simulink model "test1"  (R2017b)
settings: Solver=FixedStepAuto  StartTime=0.0  StopTime=inf  FixedStep=1e-3  RelTol=1e-3  EnableMultiTasking=on
undefined symbols (not defined in the file): D10, D11, D12, D2, D5, D8, D9, PTA0, PTA2, PTB9, PTC4, PTD0, PTD2, PTD3
libraries: frdmk64flib x12
settings Model: ExtModeTrigDuration=5  Creator=zhuh30  LastModifiedBy=Michael
settings OptimizationCC: PassReuseOutputArgsAs=Individual arguments  MaxStackSize=64
settings DebuggingCC: ParameterTunabilityLossMsg=error
settings HardwareCC: ProdBitPerPointer=32  ProdBitPerSizeT=32  ProdBitPerPtrDiffT=32  ProdLargestAtomicInteger=Long  ProdLargestAtomicFloat=Double  ProdWordSize=32  ProdHWDeviceType=ARM Compatible->ARM Cortex
settings SFSimCC: MATLABDynamicMemAlloc=off
settings RTWCC: SystemTargetFile=ert.tlc  HardwareBoard=NXP FRDM-K64F  TemplateMakefile=ert_default_tmf  GenerateReport=on  Toolchain=GNU Tools for ARM Embedded Processors  IncludeHyperlinkInReport=on  LaunchReport=on  GenerateTraceInfo=on  GenerateTraceReport=on  GenerateTraceReportSl=on  GenerateTraceReportSf=on  GenerateTraceReportEml=on
settings CodeAppCC: ForceParamTrailComments=on  IgnoreCustomStorageClasses=off  OperatorAnnotations=on  SimulinkDataObjDesc=on  SFDataObjDesc=on  InsertBlockDesc=on

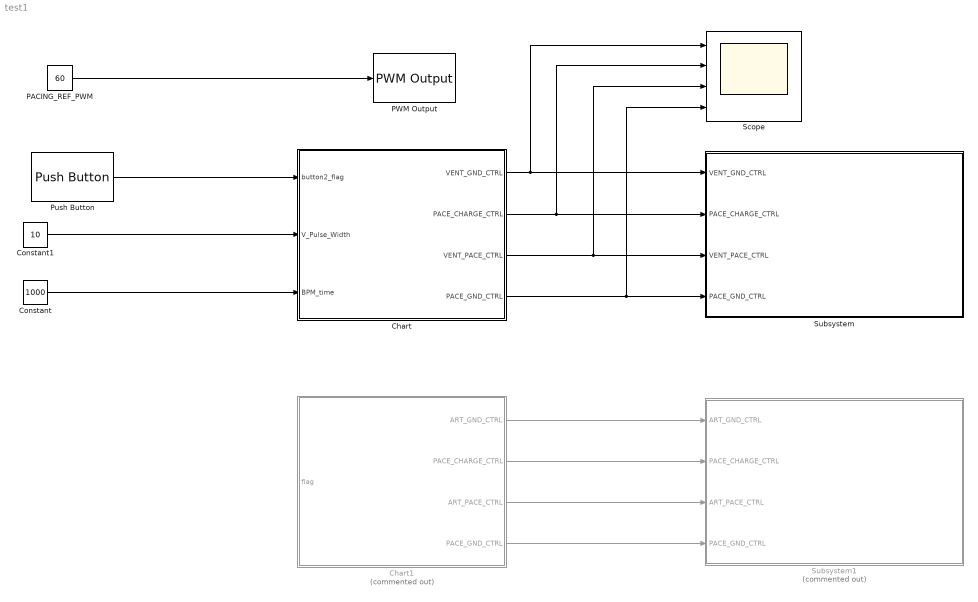
== system test1 ==
  Chart : Stateflow chart  TreatAsAtomicUnit=on
  Chart1 : Stateflow chart  Commented=on  TreatAsAtomicUnit=on
  Constant : Constant  Value=1000
  Constant1 : Constant  Value=10
  PACING_REF_PWM : Constant  Value=60  OutDataTypeStr=uint16
  PWM Output : frdmk64flib/PWM Output  Whichpin=PTA2 (D5)  InitialFrequency=1000  InitialDutyCycle=60
      settings: SourceProductName=Simulink Coder Support Package for NXP FRDM-K64F Board
  Push Button : frdmk64flib/Push Button  Whichswitch=SW2  SampleTime1=-1
      settings: SourceProductName=Simulink Coder Support Package for NXP FRDM-K64F Board
  Scope : Scope  NumInputPorts=4
  Subsystem : Subsystem
  Subsystem1 : Subsystem  Commented=on
  wires:
  Chart/2(PACE_CHARGE_CTRL) -> Scope/2, Subsystem/2(PACE_CHARGE_CTRL)
  Chart/3(VENT_PACE_CTRL) -> Scope/3, Subsystem/3(VENT_PACE_CTRL)
  Chart/4(PACE_GND_CTRL) -> Scope/4, Subsystem/4(PACE_GND_CTRL)
  PACING_REF_PWM/1 -> PWM Output/1
  Chart/1(VENT_GND_CTRL) -> Scope/1, Subsystem/1(VENT_GND_CTRL)
  Push Button/1 -> Chart/1(button2_flag)
  Chart1/4(PACE_GND_CTRL) -> Subsystem1/4(PACE_GND_CTRL)
  Chart1/2(PACE_CHARGE_CTRL) -> Subsystem1/2(PACE_CHARGE_CTRL)
  Chart1/3(ART_PACE_CTRL) -> Subsystem1/3(ART_PACE_CTRL)
  Chart1/1(ART_GND_CTRL) -> Subsystem1/1(ART_GND_CTRL)
  Constant/1 -> Chart/3(BPM_time)
  Constant1/1 -> Chart/2(V_Pulse_Width)

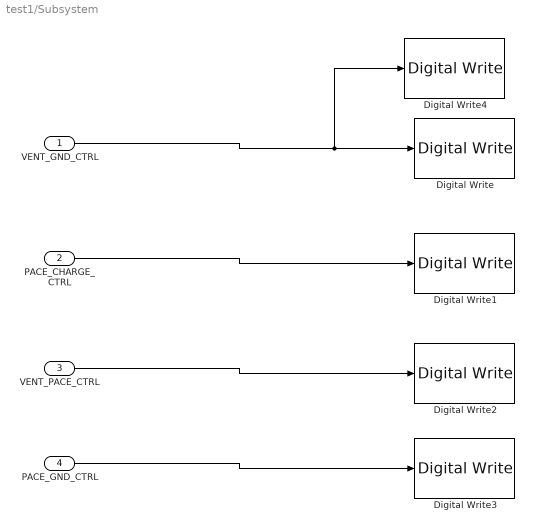
== system test1/Subsystem ==
  VENT_GND_CTRL : Inport
  PACE_CHARGE_CTRL : Inport  Port=2
  VENT_PACE_CTRL : Inport  Port=3
  PACE_GND_CTRL : Inport  Port=4
  Digital Write : frdmk64flib/Digital Write  Whichpin=PTD3 (D12)
      settings: SourceProductName=Simulink Coder Support Package for NXP FRDM-K64F Board
  Digital Write1 : frdmk64flib/Digital Write  Whichpin=PTB9 (D2)
      settings: SourceProductName=Simulink Coder Support Package for NXP FRDM-K64F Board
  Digital Write2 : frdmk64flib/Digital Write  Whichpin=PTC4 (D9)
      settings: SourceProductName=Simulink Coder Support Package for NXP FRDM-K64F Board
  Digital Write3 : frdmk64flib/Digital Write  Whichpin=PTD0 (D10)
      settings: SourceProductName=Simulink Coder Support Package for NXP FRDM-K64F Board
  Digital Write4 : frdmk64flib/Digital Write  Whichpin=RED_LED
      settings: SourceProductName=Simulink Coder Support Package for NXP FRDM-K64F Board
  wires:
  VENT_GND_CTRL/1 -> Digital Write4/1, Digital Write/1
  PACE_CHARGE_CTRL/1 -> Digital Write1/1
  VENT_PACE_CTRL/1 -> Digital Write2/1
  PACE_GND_CTRL/1 -> Digital Write3/1

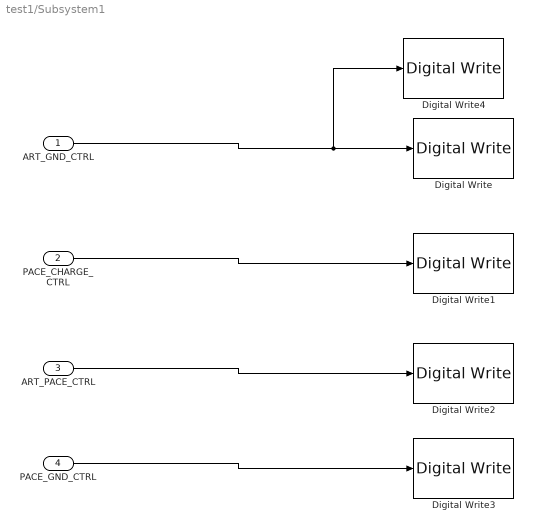
== system test1/Subsystem1 ==
  ART_GND_CTRL : Inport
  PACE_CHARGE_CTRL : Inport  Port=2
  ART_PACE_CTRL : Inport  Port=3
  PACE_GND_CTRL : Inport  Port=4
  Digital Write : frdmk64flib/Digital Write  Whichpin=PTD2 (D11)
      settings: SourceProductName=Simulink Coder Support Package for NXP FRDM-K64F Board
  Digital Write1 : frdmk64flib/Digital Write  Whichpin=PTB9 (D2)
      settings: SourceProductName=Simulink Coder Support Package for NXP FRDM-K64F Board
  Digital Write2 : frdmk64flib/Digital Write  Whichpin=PTA0 (D8)
      settings: SourceProductName=Simulink Coder Support Package for NXP FRDM-K64F Board
  Digital Write3 : frdmk64flib/Digital Write  Whichpin=PTD0 (D10)
      settings: SourceProductName=Simulink Coder Support Package for NXP FRDM-K64F Board
  Digital Write4 : frdmk64flib/Digital Write  Whichpin=RED_LED
      settings: SourceProductName=Simulink Coder Support Package for NXP FRDM-K64F Board
  wires:
  ART_GND_CTRL/1 -> Digital Write4/1, Digital Write/1
  PACE_CHARGE_CTRL/1 -> Digital Write1/1
  ART_PACE_CTRL/1 -> Digital Write2/1
  PACE_GND_CTRL/1 -> Digital Write3/1

== stateflow chart test1/Chart1 ==
  state Charging_state
    entry:
    PACE_CHARGE_CTRL = true;
    ART_PACE_CTRL = false;
    ART_GND_CTRL = true;
    PACE_GND_CTRL = true;
  state Pacing_state
    entry:
    PACE_CHARGE_CTRL = false;
    ART_PACE_CTRL = true;
    ART_GND_CTRL = false;
    PACE_GND_CTRL = true;
  Charging_state -> Pacing_state [order 1] : after(990,msec)
  (default) -> Charging_state
  Pacing_state -> Charging_state : after(10,msec)
  Charging_state -> Charging_state [order 2] : [flag == 1]
  data: ART_GND_CTRL output; PACE_CHARGE_CTRL output; ART_PACE_CTRL output; PACE_GND_CTRL output; flag input

== stateflow chart test1/Chart ==
  state Charging_state
    entry:
    PACE_CHARGE_CTRL = true;
    VENT_PACE_CTRL = false;
    VENT_GND_CTRL = true;
    PACE_GND_CTRL = true;
  state Pacing_state
    entry:
    PACE_CHARGE_CTRL = false;
    VENT_PACE_CTRL = true;
    VENT_GND_CTRL = false;
    PACE_GND_CTRL = true;
  state Delay_state
    entry:
    PACE_CHARGE_CTRL = true;
    VENT_PACE_CTRL = false;
    VENT_GND_CTRL = true;
    PACE_GND_CTRL = true;
  Charging_state -> Pacing_state [order 1] : after(BPM_time-V_Pulse_Width,msec)
  (default) -> Charging_state
  Pacing_state -> Charging_state [order 1] : after(V_Pulse_Width,msec)
  Delay_state -> Pacing_state [order 1] : after(BPM_time,msec)
  Pacing_state -> Delay_state [order 2] : [button2_flag == 1]
  Charging_state -> Delay_state [order 2] : [button2_flag == 1]
  Delay_state -> Delay_state [order 2] : [button2_flag==1]
  data: VENT_GND_CTRL output; PACE_CHARGE_CTRL output; VENT_PACE_CTRL output; PACE_GND_CTRL output; button2_flag input; V_Pulse_Width input; BPM_time input
